simulink model "tp3partie2"  (Simulink 9.2)
settings: Solver=ode45  StartTime=0.0  StopTime=2000  RelTol=1e-3  EnableMultiTasking=on
undefined symbols (not defined in the file): gama, k, k0, teta0
settings Model: Creator=AMANI  LastModifiedBy=User
settings DataIOCC: SaveFormat=StructureWithTime
settings DebuggingCC: UnderspecifiedInitializationDetection=Simplified  MergeDetectMultiDrivingBlocksExec=error  StateNameClashWarn=none
settings HardwareCC: ProdIntDivRoundTo=Zero  ProdEndianess=LittleEndian  ProdHWDeviceType=Specified
settings GRTTargetCC: GeneratePreprocessorConditionals=Use local settings
settings ConfigComp: CovExternalEMLEnable=on

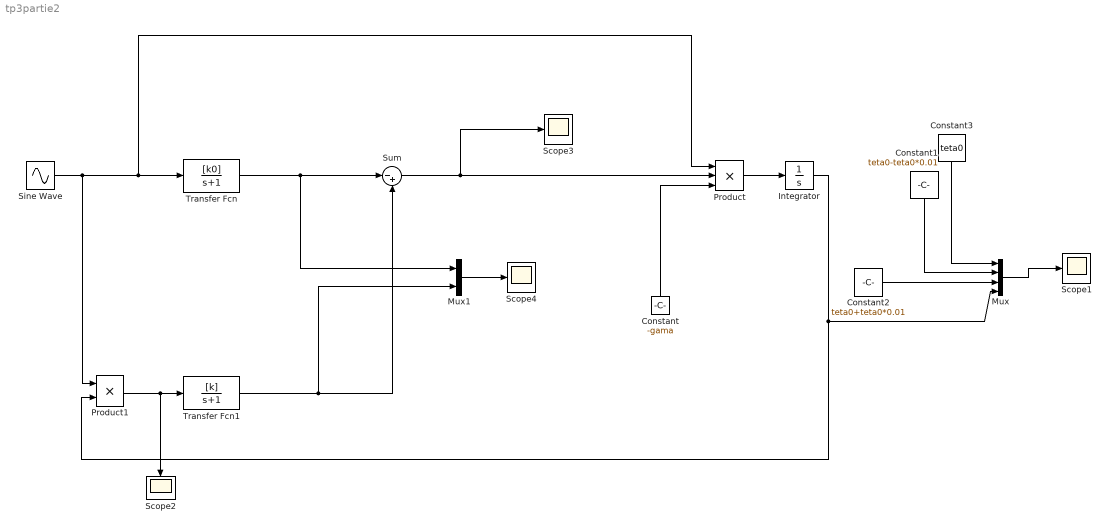
== system tp3partie2 ==
  Constant : Constant  Value=-gama
  Constant1 : Constant  Value=teta0-teta0*0.01
  Constant2 : Constant  Value=teta0+teta0*0.01
  Constant3 : Constant  Value=teta0
  Integrator : Integrator
  Mux : Mux
  Mux1 : Mux  Inputs=2
  Product : Product  Inputs=3
  Product1 : Product
  Scope{1..4} (4 alike) : Scope
  Sine Wave : Sin  SampleTime=0
  Sum : Sum  Inputs=|-+
  Transfer Fcn : TransferFcn  Numerator=[k0]  Denominator=[1 1]
  Transfer Fcn1 : TransferFcn  Numerator=[k]  Denominator=[1 1]
  wires:
  Transfer Fcn1/1 -> Mux1/2, Sum/2
  Sum/1 -> Scope3/1, Product/2
  Transfer Fcn/1 -> Mux1/1, Sum/1
  Product/1 -> Integrator/1
  Integrator/1 -> Product1/2, Mux/4
  Constant/1 -> Product/3
  Product1/1 -> Scope2/1, Transfer Fcn1/1
  Mux/1 -> Scope1/1
  Constant1/1 -> Mux/2
  Constant2/1 -> Mux/3
  Constant3/1 -> Mux/1
  Sine Wave/1 -> Product1/1, Product/1, Transfer Fcn/1
  Mux1/1 -> Scope4/1
